simulink model "gm_working_motor"  (R2017a)
settings: Solver=FixedStepAuto  StartTime=0.0  StopTime=inf  RelTol=1e-3  EnableMultiTasking=on
libraries: simulink x3, hdlsllib x3
settings Model: Creator=hyang344  LastModifiedBy=hyang344
settings SolverCC: AutoInsertRateTranBlk=on
settings OptimizationCC: BlockReduction=off  ConditionallyExecuteInputs=off  DefaultParameterBehavior=Inlined
settings DebuggingCC: AlgebraicLoopMsg=error  InheritedTsInSrcMsg=none  SingleTaskRateTransMsg=error
settings HardwareCC: ProdBitPerPointer=32  ProdBitPerSizeT=32  ProdBitPerPtrDiffT=32  ProdLargestAtomicFloat=None  ProdIntDivRoundTo=Undefined  ProdEndianess=Unspecified  ProdWordSize=32  ProdHWDeviceType=ASIC/FPGA->ASIC/FPGA  ProdEqTarget=off

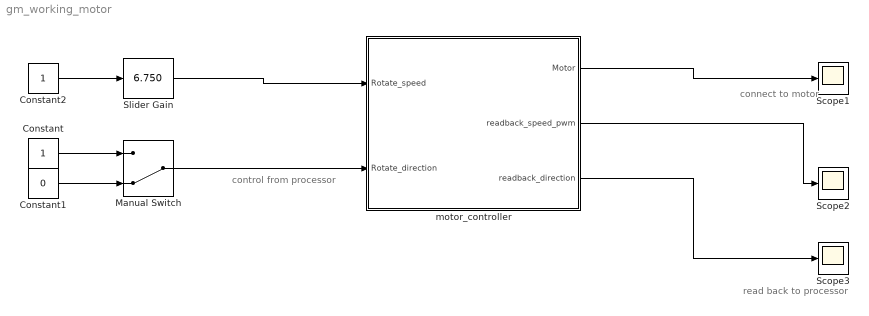
== system gm_working_motor ==
  note: read back to
      | processor
  note: connect to
      | motor
  note: control from
      | processor
  Constant : Constant  OutDataTypeStr=boolean
  Constant1 : Constant  Value=0  OutDataTypeStr=boolean
  Constant2 : Constant  OutDataTypeStr=fixdt(0, 4, 0)  SampleTime=0.1
  Manual Switch : ManualSwitch  CurrentSetting=0
  Scope1 : Scope
  Scope2 : Scope
  Scope3 : Scope
  Slider Gain : simulink/Math Operations/Slider Gain  gain=6.750  low=0  high=15
  motor_controller : Subsystem  TreatAsAtomicUnit=on
  wires:
  motor_controller/3("readback_direction ") -> Scope3/1
  motor_controller/2(readback_speed_pwm) -> Scope2/1
  Manual Switch/1 -> motor_controller/2(Rotate_direction)
  Constant/1 -> Manual Switch/1
  motor_controller/1(Motor) -> Scope1/1
  Constant2/1 -> Slider Gain/1
  Slider Gain/1 -> motor_controller/1(Rotate_speed)
  Constant1/1 -> Manual Switch/2

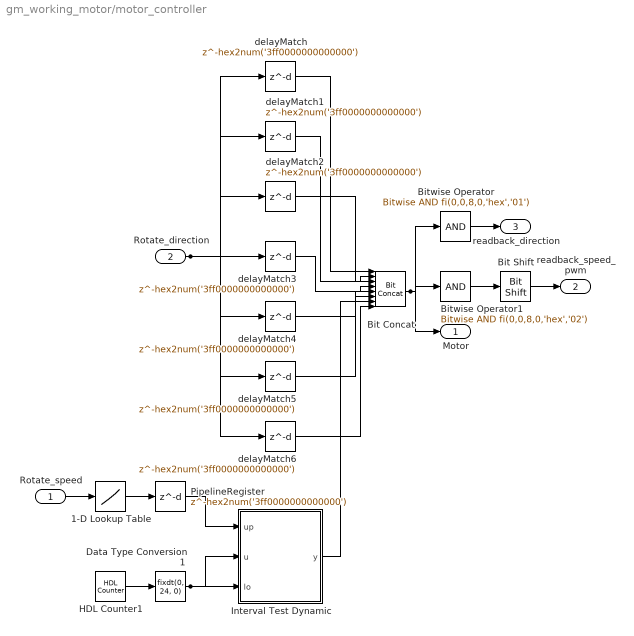
== system gm_working_motor/motor_controller ==
  Rotate_speed : Inport  OutDataTypeStr=fixdt(0, 4, 0)  SampleTime=0.1
  Rotate_direction : Inport  Port=2  OutDataTypeStr=boolean  SampleTime=0.1
  1-D Lookup Table : Lookup_n-D  NumberOfTableDimensions=1  BreakpointsForDimension1=[fi(0,0,4,0,'hex','0') fi(0,0,4,0,'hex','1') fi(0,0,4,0,'hex','2') fi(0,0,4,0,'hex','3') fi(0,0,4,0,'hex','4') fi(0,0,4,0,'hex','5') fi(0,0,4,0,'hex','6') fi(0,0,4,0,'hex','7') fi(0,0,4,0,'hex','8') fi(0,0,4,0,'hex','9') fi(0,0,4,0,'hex','a') fi(0,0,4,0,'hex','b') fi(0,0,4,0,'hex','c') fi(0,0,4,0,'hex','d') fi(0,0,4,0,'hex','e') fi(0,0,4,0,'hex','f')]  Table="reshape([fi(0,0,24,0,'hex','00186a') fi(0,0,24,0,'hex','001d4c') fi(0,0,24,0,'hex','00222e') fi(0,0,24,0,'hex','002710') fi(0,0,24,0,'hex','002bf2') fi(0,0,24,0,'hex','0030d4') fi(0,0,24,0,'hex','0035b6') fi(0,0,24,0,'hex','003a98') fi(0,0,24,0,'hex','003f7a') fi(0,0,24,0,'hex','00445c') fi(0,0,24,0,'hex','00493e') fi(0,0,24,0,'hex','004e20') fi(0,0,24,0,'hex','005302') fi(0,0,24,0,'hex','0057e4') fi(0,0,24,0,'hex','005cc6') fi(0,0,24,0,'hex','0061a8')].', [1  16])"  InterpMethod=Flat  DiagnosticForOutOfRangeInput=Error  SampleTime=0.1  OutDataTypeStr=fixdt(0, 24, 0)  RndMeth=Simplest  InputSameDT=on
  Bit Concat : hdlsllib/HDL Operations/Bit Concat  numInputs=8
      settings: SourceProductName=HDL Coder  SourceProductBaseCode=HD
  Bit Shift : hdlsllib/HDL Operations/Bit Shift  mode=Shift Right Logical  N=hex2num('3ff0000000000000')
      settings: SourceProductName=HDL Coder  SourceProductBaseCode=HD
  Bitwise Operator : simulink/Logic and Bit Operations/Bitwise Operator  logicop=AND  UseBitMask=on  BitMask=fi(0,0,8,0,'hex','01')  BitMaskRealWorld=Real World Value
  Bitwise Operator1 : simulink/Logic and Bit Operations/Bitwise Operator  logicop=AND  UseBitMask=on  BitMask=fi(0,0,8,0,'hex','02')  BitMaskRealWorld=Real World Value
  Data Type Conversion1 : DataTypeConversion  OutDataTypeStr=fixdt(0, 24, 0)  SampleTime=0.1
  HDL Counter1 : hdlsllib/HDL Operations/HDL Counter  CountType=Count limited  CountInit=hex2num('0000000000000000')  CountStep=hex2num('3ff0000000000000')  CountMax=hex2num('40d86a0000000000')  CountFromType=Initial value  CountFrom=hex2num('0000000000000000')  CountResetPort=off  CountLoadPort=off  CountEnbPort=off  CountDirPort=off  CountDataType=Unsigned  CountWordLen=16  CountFracLen=0  CountSampTime=0.1
      settings: SourceProductName=HDL Coder  SourceProductBaseCode=HD
  Interval Test Dynamic : Subsystem  mask(Interval Test Dynamic){IntervalClosedRight=on, IntervalClosedLeft=on, OutDataTypeStr=boolean}
      mask prompts: IntervalClosedRight "Simulink:masks:IntervalClosedOnRight_MP"; IntervalClosedLeft "Simulink:masks:IntervalClosedOnLeft_MP"; OutDataTypeStr "Simulink:masks:OutputDataType_MP"
      mask help: Simulink:masks:IntervalTest_MD
      mask TypeOptions OutDataTypeStr: Simulink:masks:uint8 | Simulink:masks:boolean
  PipelineRegister : Delay  DelayLength=hex2num('3ff0000000000000')  InitialCondition=0  InputProcessing=Inherited  SampleTime=0.1
  delayMatch{,1..6} (7 alike) : Delay  DelayLength=hex2num('3ff0000000000000')  InitialCondition=0  InputProcessing=Inherited  SampleTime=0.1
  Motor : Outport
  readback_speed_pwm : Outport  Port=2
  "readback_direction " : Outport  Port=3
  wires:
  Rotate_speed/1 -> 1-D Lookup Table/1
  delayMatch/1 -> Bit Concat/1
  PipelineRegister/1 -> Interval Test Dynamic/1(up)
  Bit Concat/1 -> Bitwise Operator1/1, Bitwise Operator/1, Motor/1
  Bit Shift/1 -> readback_speed_pwm/1
  Bitwise Operator/1 -> "readback_direction "/1
  Bitwise Operator1/1 -> Bit Shift/1
  Data Type Conversion1/1 -> Interval Test Dynamic/3(lo), Interval Test Dynamic/2(u)
  HDL Counter1/1 -> Data Type Conversion1/1
  Interval Test Dynamic/1(y) -> Bit Concat/7
  delayMatch1/1 -> Bit Concat/2
  delayMatch2/1 -> Bit Concat/3
  delayMatch3/1 -> Bit Concat/4
  delayMatch4/1 -> Bit Concat/5
  delayMatch5/1 -> Bit Concat/6
  delayMatch6/1 -> Bit Concat/8
  Rotate_direction/1 -> delayMatch6/1, delayMatch5/1, delayMatch4/1, delayMatch3/1, delayMatch2/1, delayMatch1/1, delayMatch/1
  1-D Lookup Table/1 -> PipelineRegister/1

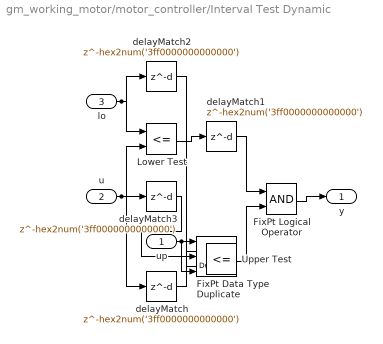
== system gm_working_motor/motor_controller/Interval Test Dynamic ==
  up : Inport  OutDataTypeStr=fixdt(0, 24, 0)  SampleTime=0.1
  u : Inport  Port=2  OutDataTypeStr=fixdt(0, 24, 0)  SampleTime=0.1
  lo : Inport  Port=3  OutDataTypeStr=fixdt(0, 24, 0)  SampleTime=0.1
  FixPt Data Type Duplicate : DataTypeDuplicate  DisableCoverage=on  NumInputPorts=3
  FixPt Logical Operator : Logic  AllPortsSameDT=off  OutDataTypeStr=boolean  SampleTime=0.1
  Lower Test : RelationalOperator  Operator=<=  OutDataTypeStr=boolean  SampleTime=0.1  RndMeth=Nearest
  Upper Test : RelationalOperator  Operator=<=  OutDataTypeStr=boolean  SampleTime=0.1  RndMeth=Nearest
  delayMatch{,1..3} (4 alike) : Delay  DelayLength=hex2num('3ff0000000000000')  InitialCondition=0  InputProcessing=Inherited  SampleTime=0.1
  y : Outport
  wires:
  delayMatch/1 -> Upper Test/1
  delayMatch2/1 -> FixPt Data Type Duplicate/1
  FixPt Logical Operator/1 -> y/1
  delayMatch1/1 -> FixPt Logical Operator/1
  Upper Test/1 -> FixPt Logical Operator/2
  up/1 -> Upper Test/2, FixPt Data Type Duplicate/3
  u/1 -> delayMatch3/1, delayMatch/1, Lower Test/2
  lo/1 -> delayMatch2/1, Lower Test/1
  delayMatch3/1 -> FixPt Data Type Duplicate/2
  Lower Test/1 -> delayMatch1/1
